simulink model "Inverse_dynamic_regulation"  (R2019b)
settings: Solver=VariableStepAuto  StartTime=0.0  StopTime=10  FixedStep=.001  MaxStep=.1  RelTol=1e-3
settings Model: Creator=imi  LastModifiedBy=Ali Alaei
settings DataIOCC: ReturnWorkspaceOutputs=off
settings DebuggingCC: ArithmeticOperatorsInVariantConditions=warning
settings SFSimCC: SimUseLocalCustomCode=off  CustomCodeUndefinedFunction=UseInterfaceOnly
settings RTWCC: RTWUseLocalCustomCode=off
settings CodeAppCC: StateflowObjectComments=on

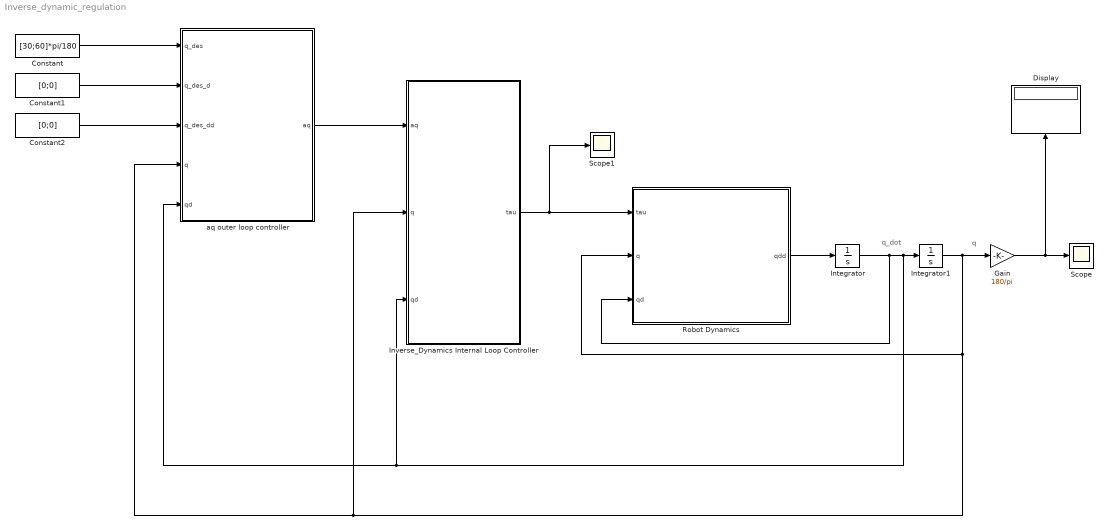
== system Inverse_dynamic_regulation ==
  note: q
  note: q_dot
  Constant : Constant  Value=[30;60]*pi/180
  Constant1 : Constant  Value=[0;0]
  Constant2 : Constant  Value=[0;0]
  Display : Display
  Gain : Gain  Gain=180/pi
  Integrator : Integrator  InitialCondition=zeros(2,1)
  Integrator1 : Integrator  InitialCondition=[45;95]*pi/180*0
  Inverse_Dynamics Internal Loop Controller : MATLAB Function  TreatAsAtomicUnit=on
  Robot Dynamics : MATLAB Function  TreatAsAtomicUnit=on
  Scope : Scope
  Scope1 : Scope
  aq outer loop controller : MATLAB Function  TreatAsAtomicUnit=on
  wires:
  Integrator/1 -> aq outer loop controller/5(qd), Inverse_Dynamics Internal Loop Controller/3(qd), Integrator1/1, Robot Dynamics/3(qd)
  Robot Dynamics/1(qdd) -> Integrator/1
  Integrator1/1 -> aq outer loop controller/4(q), Inverse_Dynamics Internal Loop Controller/2(q), Robot Dynamics/2(q), Gain/1
  Inverse_Dynamics Internal Loop Controller/1(tau) -> Scope1/1, Robot Dynamics/1(tau)
  Gain/1 -> Scope/1, Display/1
  Constant/1 -> aq outer loop controller/1(q_des)
  Constant1/1 -> aq outer loop controller/2(q_des_d)
  Constant2/1 -> aq outer loop controller/3(q_des_dd)
  aq outer loop controller/1(aq) -> Inverse_Dynamics Internal Loop Controller/1(aq)

== matlab function Inverse_dynamic_regulation/Inverse_Dynamics Internal Loop Controller ==
  data: aq input; q input; qd input; tau output
function tau = fcn(aq,q,qd)

q1=q(1);
q2=q(2);

q1d=qd(1);
q2d=qd(2);



m1=2;
m2=1.4;

I1=.5;
I2=.1;

l1=.8;
l2=.8;

lc1=.4;
lc2=.4;


g=9.81;



d11=m1*lc1^2+I1+I2+m2*(l1^2+lc2^2+2*l1*lc2*cos(q2));
d12=m2*lc2^2+I2+m2*l2*lc2*cos(q2);
d21=m2*lc2^2+I2+m2*l2*lc2*cos(q2);
d22=m2*lc2^2+I2;

c11=-m2*l1*lc2*sin(q2)*q2d;
c12=-m2*l1*lc2*sin(q2)*(q1d+q2d);
c21=m2*l1*lc2*sin(q2)*q1d;
c22=0;

g11=m1*lc1*g*cos(q1)+m2*g*(lc2*cos(q1+q2)+l1*cos(q1));
g21=m2*lc2*g*cos(q1+q2);


M=[d11,d12;d21,d22];
C=[c11 c12;c21 c22];
G=[g11;g21];



tau=M*aq+C*qd+G;

== matlab function Inverse_dynamic_regulation/Robot Dynamics ==
  data: tau input; q input; qdd output; qd input
function qdd = fcn(tau,q,qd)

q1=q(1);
q2=q(2);

q1d=qd(1);
q2d=qd(2);



m1=2;
m2=1.4;

I1=.5;
I2=.1;

l1=.8;
l2=.8;

lc1=.4;
lc2=.4;


g=9.81;



d11=m1*lc1^2+I1+I2+m2*(l1^2+lc2^2+2*l1*lc2*cos(q2));
d12=m2*lc2^2+I2+m2*l2*lc2*cos(q2);
d21=m2*lc2^2+I2+m2*l2*lc2*cos(q2);
d22=m2*lc2^2+I2;

c11=-m2*l1*lc2*sin(q2)*q2d;
c12=-m2*l1*lc2*sin(q2)*(q1d+q2d);
c21=m2*l1*lc2*sin(q2)*q1d;
c22=0;

g11=m1*lc1*g*cos(q1)+m2*g*(lc2*cos(q1+q2)+l1*cos(q1));
g21=m2*lc2*g*cos(q1+q2);



M=[d11,d12;d21,d22];
C=[c11 c12;c21 c22];
G=[g11;g21];



qdd=pinv(M)*(tau-C*qd-G);

== matlab function Inverse_dynamic_regulation/aq outer loop controller ==
  data: q_des input; q_des_d input; q_des_dd input; q input; qd input; aq output
function aq = fcn(q_des,q_des_d,q_des_dd,q,qd)

q1=q(1);
q2=q(2);

q1d=qd(1);
q2d=qd(2);




q_tilde=q-q_des;
q_tilde_d=qd-q_des_d;


zita=1;
wn=2*pi*3;

K1=eye(2)*2*zita*wn;
K0=eye(2)*wn^2;


aq=q_des_dd-K0*q_tilde-K1*q_tilde_d;%external loop
